simulink model "zero_to_hero_sect1to5"  (R2023a)
settings: Solver=VariableStepAuto  StartTime=0.0  StopTime=runtime  FixedStep=0.01  MaxStep=0.01  RelTol=1e-3
undefined symbols (not defined in the file): b, F, k, m
libraries: simulink x1
settings Model: Creator=fycce  LastModifiedBy=fycce
settings DataIOCC: SaveOutput=off  SaveTime=off  ReturnWorkspaceOutputs=off

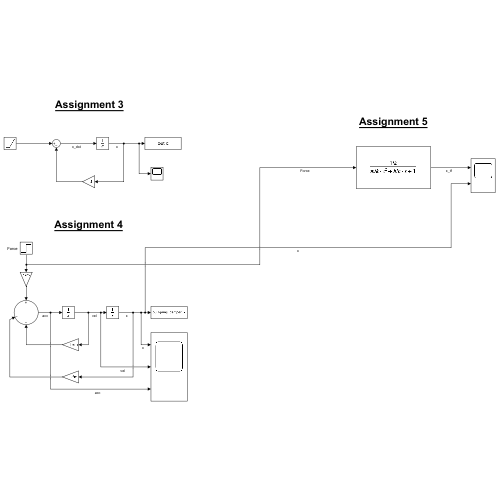
[thumbnail: Simulink's stored preview of the top-level diagram]
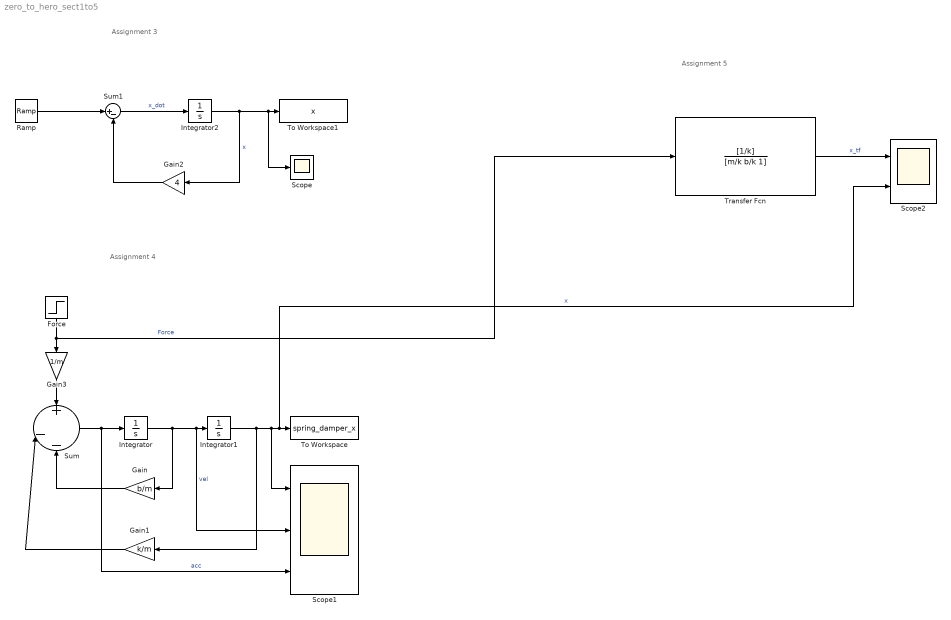
== system zero_to_hero_sect1to5 ==
  note: Assignment 4
  note: Assignment 3
  note: Assignment 5
  Force : Step  After=F  SampleTime=0
  Gain : Gain  Gain=b/m
  Gain1 : Gain  Gain=k/m
  Gain2 : Gain  Gain=4
  Gain3 : Gain  Gain=1/m
  Integrator : Integrator
  Integrator1 : Integrator
  Integrator2 : Integrator
  Ramp : simulink/Sources/Ramp  slope=1  start=0  InitialOutput=0
  Scope : Scope
  Scope1 : Scope  NumInputPorts=3
  Scope2 : Scope  NumInputPorts=2
  Sum : Sum  Inputs=+||||-||-
  Sum1 : Sum  Inputs=|+-
  To Workspace : ToWorkspace  VariableName=spring_damper_x  SaveFormat=Timeseries  SampleTime=-1
  To Workspace1 : ToWorkspace  VariableName=x  SaveFormat=Timeseries  SampleTime=-1
  Transfer Fcn : TransferFcn  Numerator=[1/k]  Denominator=[m/k b/k 1]
  wires:
  Sum/1 -> Integrator/1, Scope1/3  "acc"
  Integrator/1 -> Gain/1, Scope1/2, Integrator1/1  "vel"
  Integrator1/1 -> Gain1/1, Scope1/1, Scope2/2, To Workspace/1  "x"
  Gain/1 -> Sum/3
  Gain1/1 -> Sum/2
  Integrator2/1 -> Gain2/1, Scope/1, To Workspace1/1  "x"
  Gain2/1 -> Sum1/2
  Sum1/1 -> Integrator2/1  "x_dot"
  Ramp/1 -> Sum1/1
  Transfer Fcn/1 -> Scope2/1  "x_tf"
  Force/1 -> Gain3/1, Transfer Fcn/1  "Force"
  Gain3/1 -> Sum/1
